simulink model "DCDC_boost_converter"  (R2017a)
settings: Solver=ode23tb  StartTime=0.0  StopTime=1.5  MaxStep=1e-6  RelTol=1e-3
undefined symbols (not defined in the file): C, Cd, L, Ro
libraries: powerlib x10, powerlib_meascontrol x1
settings Model: Creator=Marcos  LastModifiedBy=Marcos

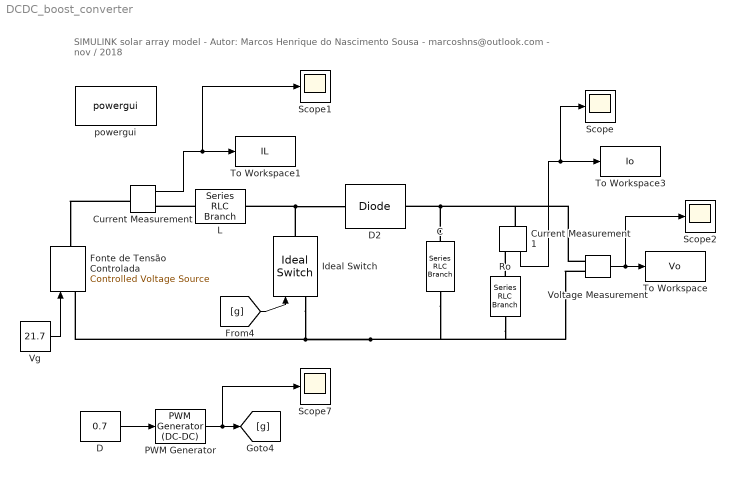
== system DCDC_boost_converter ==
  note: SIMULINK solar array model - Autor: Marcos Henrique do Nascimento Sousa - marcoshns@outlook.com - nov / 2018
  C : powerlib/Elements/Series RLC Branch  LConnTagsString=__new0  RConnTagsString=__new0  BranchType=C  Resistance=1  Inductance=1e-3  SetiL0=off  InitialCurrent=0  Capacitance=C  Setx0=on  InitialVoltage=0  Measurements=None
  Current Measurement : powerlib/Measurements/Current Measurement  PhasorSimulation=off  OutputType=Complex  PSBequivalent=0
  Current Measurement1 : powerlib/Measurements/Current Measurement  PhasorSimulation=off  OutputType=Complex  PSBequivalent=0
  D : Constant  Value=0.7
  D2 : powerlib/Power Electronics/Diode  Ron=0.00001  Lon=0  Vf=0  IC=0  UseSnubber=0  Rs=500  Cs=250e-9  Measurements=off
  Fonte de Tensão Controlada : powerlib/Electrical Sources/Controlled Voltage Source  Initialize=on  Source_Type=AC  Amplitude=0  Phase=0  Frequency=0  Measurements=None
  Ideal Switch : powerlib/Power Electronics/Ideal Switch  Ron=0.001  Lon=0  IC=0  Rs=1e5  Cs=inf  Measurements=off
  L : powerlib/Elements/Series RLC Branch  LConnTagsString=__new0  RConnTagsString=__new0  BranchType=L  Resistance=1  Inductance=L  SetiL0=on  InitialCurrent=0  Capacitance=1e-6  Setx0=off  InitialVoltage=0  Measurements=None
  "PWM Generator " : powerlib_meascontrol/Pulse & Signal Generators/PWM Generator (DC-DC)  Fsw=10000  Ts=0
  Ro : powerlib/Elements/Series RLC Branch  LConnTagsString=__new0  RConnTagsString=__new0  BranchType=R  Resistance=Ro  Inductance=L  SetiL0=on  InitialCurrent=0  Capacitance=Cd  Setx0=off  InitialVoltage=0  Measurements=None
  Scope{,1..2,7} (4 alike) : Scope
  To Workspace : ToWorkspace  VariableName=Vo  SampleTime=-1
  To Workspace1 : ToWorkspace  VariableName=IL  SampleTime=-1
  To Workspace3 : ToWorkspace  VariableName=Io  SampleTime=-1
  Vg : Constant  Value=21.7
  Voltage Measurement : powerlib/Measurements/Voltage Measurement  PhasorSimulation=off  OutputType=Complex  PSBequivalent=0
  powergui : powerlib/powergui  Priority=1  SimulationMode=Discrete  SampleTime=1e-6  frequency=60  Iterations=50  frequencyindice=0  Pbase=100e6  ErrMax=1e-4  UnitsV=kV  UnitsW=MW  buscounter=0  FunctionMessages=off  echomessages=off  EnableUseOfTLC=off  CurrentSourceSwitches=off  DisableSnubberDevices=off  DisableRonSwitches=off  DisableVfSwitches=off  DisplayEquations=off  SolverType=Tustin/Backward Euler (TBE)  Interpol=off  ExternalGateDelay=off  methode=off  Ts=100  x0status=blocks  SPID=on  SwTol=0  HookPort=off  RestoreLinks=warning  ResistiveCurrentMeasurement=off  Frange=[0:2:500]  Ylog=off  Xlog=on  ShowGrid=off  save=off  variable=ZData  structure=0  ZoomFFT=off  StartTime=0.0  cycles=1  DisplayStyle=1  fundamental=60  FreqAxis=off  MaxFrequency=1000  frequencyindicesteady=1  RmsSteady=1  display=off
  wires:
  [g] -> Ideal Switch/1
  Vg/1 -> Fonte de Tensão Controlada/1
  Voltage Measurement/1 -> Scope2/1, To Workspace/1
  "PWM Generator "/1 -> Scope7/1, [g]
  D/1 -> "PWM Generator "/1
  Current Measurement/1 -> Scope1/1, To Workspace1/1
  Current Measurement1/1 -> Scope/1, To Workspace3/1
  connections:
  Current Measurement/LConn1 -- Fonte de Tensão Controlada/RConn1
  C/LConn1 -- Voltage Measurement/LConn1 -- Current Measurement1/LConn1 -- D2/RConn1
  Ro/RConn1 -- Voltage Measurement/LConn2 -- C/RConn1 -- Fonte de Tensão Controlada/LConn1 -- Ideal Switch/LConn1
  L/LConn1 -- Current Measurement/RConn1
  Ideal Switch/RConn1 -- L/RConn1 -- D2/LConn1
  Ro/LConn1 -- Current Measurement1/RConn1
